simulink model "testSerializedParamsNew"  (R2014a)
settings: Solver=FixedStepDiscrete  StartTime=0.0  StopTime=Inf  FixedStep=0.001  RelTol=1e-3
undefined symbols (not defined in the file or in its folder): SimulinkParameter_TestParam, SimulinkParameter_TestParamPulse, SimulinkParameter_TestParamToggle, SimulinkParameter_TunableTaskControl
libraries: slrtlib x9, dspindex x1
settings Model: SimulationMode=external  BufferReuse=off  Creator=shenoylab  LastModifiedBy=shenoylab
settings SolverCC: EnableConcurrentExecution=on
settings DataIOCC: SignalLoggingSaveFormat=ModelDataLogs
settings OptimizationCC: BlockReduction=off  OptimizeBlockIOStorage=off  BufferReuse=off  GlobalBufferReuse=off  ExpressionFolding=off  LocalBlockOutputs=off
settings DebuggingCC: MultiTaskDSMMsg=warning  MultiTaskCondExecSysMsg=none  StateNameClashWarn=warning
settings HardwareCC: ProdIntDivRoundTo=Zero  ProdEndianess=LittleEndian  ProdHWDeviceType=Generic->32-bit x86 compatible
settings RTWCC: SystemTargetFile=slrt.tlc  TemplateMakefile=slrt_default_tmf  Description=Simulink Real-Time  GenerateReport=on  ProcessScript=slrt_make_rtw_hook  LaunchReport=on  IncludeERTFirstTime=on  RTWCompilerOptimization=On
settings CodeAppCC: MATLABSourceComments=on
settings SimulinkRealTimeCC: GeneratePreprocessorConditionals=Disable all  EnableShiftOperators=on

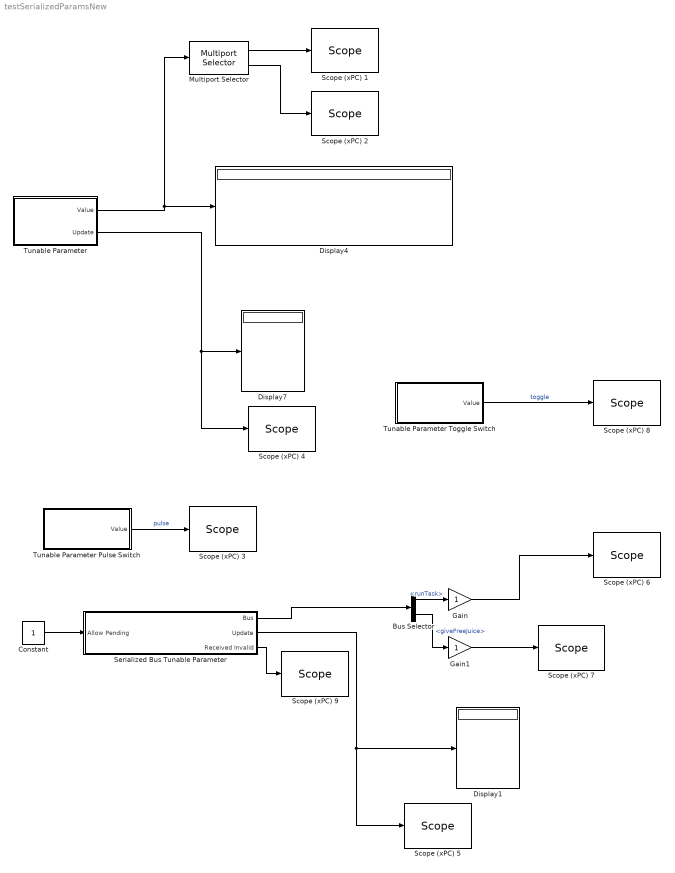
== system testSerializedParamsNew ==
  Bus Selector : BusSelector  OutputSignals=runTask,giveFreeJuice
  Constant : Constant  OutDataTypeStr=uint8
  Display1 : Display
  Display4 : Display
  Display7 : Display
  Gain : Gain  OutDataTypeStr=double
  Gain1 : Gain  OutDataTypeStr=double
  Multiport Selector : dspindex/Multiport Selector  rowsOrCols=Rows  idxCellArray={ 1, 2 }  idxErrMode=Clip Index
  Scope (xPC) 1 : slrtlib/Displays and Logging/Scope   scopeno=1  scopetype=Target  autostart=on  viewmode=Numerical  formatstr='%15.6f'  grid=on  ylimits=[0,0]  nosamples=250  noprepostsamples=0  interleave=1  triggermode=FreeRun  triggersignal=1  trigsignalfromport=off  triggerlevel=0.0  triggerslope=Either  triggerscope=1  triggersample=0  filename=data.dat  mode=Lazy  writesize=512  autorestart=off  dynamicfilemode=off  maxwritefilesize=512*1024^2
  Scope (xPC) 2 : slrtlib/Displays and Logging/Scope   scopeno=2  scopetype=Target  autostart=on  viewmode=Numerical  formatstr='%15.6f'  grid=on  ylimits=[0,0]  nosamples=250  noprepostsamples=0  interleave=1  triggermode=FreeRun  triggersignal=1  trigsignalfromport=off  triggerlevel=0.0  triggerslope=Either  triggerscope=1  triggersample=0  filename=data.dat  mode=Lazy  writesize=512  autorestart=off  dynamicfilemode=off  maxwritefilesize=512*1024^2
  Scope (xPC) 3 : slrtlib/Displays and Logging/Scope   scopeno=3  scopetype=Target  autostart=on  viewmode=Graphical rolling  formatstr='%15.6f'  grid=on  ylimits=[-1,2]  nosamples=500  noprepostsamples=0  interleave=1  triggermode=FreeRun  triggersignal=1  trigsignalfromport=off  triggerlevel=0.0  triggerslope=Either  triggerscope=1  triggersample=0  filename=data.dat  mode=Lazy  writesize=512  autorestart=off  dynamicfilemode=off  maxwritefilesize=512*1024^2
  Scope (xPC) 4 : slrtlib/Displays and Logging/Scope   scopeno=5  scopetype=Target  autostart=on  viewmode=Graphical rolling  formatstr='%15.6f'  grid=on  ylimits=[-1,2]  nosamples=500  noprepostsamples=0  interleave=1  triggermode=FreeRun  triggersignal=1  trigsignalfromport=off  triggerlevel=0.0  triggerslope=Either  triggerscope=1  triggersample=0  filename=data.dat  mode=Lazy  writesize=512  autorestart=off  dynamicfilemode=off  maxwritefilesize=512*1024^2
  Scope (xPC) 5 : slrtlib/Displays and Logging/Scope   scopeno=4  scopetype=Target  autostart=on  viewmode=Graphical rolling  formatstr='%15.6f'  grid=on  ylimits=[-1,2]  nosamples=500  noprepostsamples=0  interleave=1  triggermode=FreeRun  triggersignal=1  trigsignalfromport=off  triggerlevel=0.0  triggerslope=Either  triggerscope=1  triggersample=0  filename=data.dat  mode=Lazy  writesize=512  autorestart=off  dynamicfilemode=off  maxwritefilesize=512*1024^2
  Scope (xPC) 6 : slrtlib/Displays and Logging/Scope   scopeno=6  scopetype=Target  autostart=on  viewmode=Graphical rolling  formatstr='%15.6f'  grid=on  ylimits=[-1,2]  nosamples=250  noprepostsamples=0  interleave=1  triggermode=FreeRun  triggersignal=1  trigsignalfromport=off  triggerlevel=0.0  triggerslope=Either  triggerscope=1  triggersample=0  filename=data.dat  mode=Lazy  writesize=512  autorestart=off  dynamicfilemode=off  maxwritefilesize=512*1024^2
  Scope (xPC) 7 : slrtlib/Displays and Logging/Scope   scopeno=7  scopetype=Target  autostart=on  viewmode=Graphical rolling  formatstr='%15.6f'  grid=on  ylimits=[-1,2]  nosamples=500  noprepostsamples=0  interleave=1  triggermode=FreeRun  triggersignal=1  trigsignalfromport=off  triggerlevel=0.0  triggerslope=Either  triggerscope=1  triggersample=0  filename=data.dat  mode=Lazy  writesize=512  autorestart=off  dynamicfilemode=off  maxwritefilesize=512*1024^2
  Scope (xPC) 8 : slrtlib/Displays and Logging/Scope   scopeno=8  scopetype=Target  autostart=on  viewmode=Graphical rolling  formatstr='%15.6f'  grid=on  ylimits=[-1,2]  nosamples=500  noprepostsamples=0  interleave=1  triggermode=FreeRun  triggersignal=1  trigsignalfromport=off  triggerlevel=0.0  triggerslope=Either  triggerscope=1  triggersample=0  filename=data.dat  mode=Lazy  writesize=512  autorestart=off  dynamicfilemode=off  maxwritefilesize=512*1024^2
  Scope (xPC) 9 : slrtlib/Displays and Logging/Scope   scopeno=9  scopetype=Target  autostart=on  viewmode=Graphical rolling  formatstr='%15.6f'  grid=on  ylimits=[-1,2]  nosamples=500  noprepostsamples=0  interleave=1  triggermode=FreeRun  triggersignal=1  trigsignalfromport=off  triggerlevel=0.0  triggerslope=Either  triggerscope=1  triggersample=0  filename=data.dat  mode=Lazy  writesize=512  autorestart=off  dynamicfilemode=off  maxwritefilesize=512*1024^2
  Serialized Bus Tunable Parameter : Subsystem  AncestorBlock=libBusSerialize/Serialized Bus Tunable Parameter  mask(BusSerialize Tunable Parameter Block){paramName='TunableTaskControl'}
      mask prompts: paramName "Parameter Name"
      mask help: This block provides the value of a tunable Simulink.Parameter into the model. Since tunable parameters with xPC target can only be doubles, the functions BusSerialize.createTunableParameter and BusSerialize.setTunableParameter automatically handle typecasting and update counter insertion, and this block handles update detection, typecasting, and reshaping back to the original form. Currently, variable size parameters are not supported.
      mask init:
      | BusSerialize.maskSerializedBusTunableParameterBlockUpdate(gcb);
      mask Display:
      | port_label('output', 1, paramName);
      | port_label('output', 2, 'Update');
      | port_label('output', 3, 'Received Invalid');
      | port_label('input', 1, 'Allow Pending');
  Tunable Parameter : Subsystem  AncestorBlock=libBusSerialize/Tunable Parameter  mask(BusSerialize Tunable Parameter Block){paramName='TestParam'}
      mask prompts: paramName "Parameter Name"
      mask help: This block provides the value of a tunable Simulink.Parameter into the model. Since tunable parameters with xPC target can only be doubles, the functions BusSerialize.createTunableParameter and BusSerialize.setTunableParameter automatically handle typecasting and update counter insertion, and this block handles update detection, typecasting, and reshaping back to the original form. Currently, variable size parameters are not supported.
      mask init:
      | BusSerialize.maskTunableParameterBlockUpdate(gcb);
      mask Display:
      | port_label('output', 1, paramName)
      | port_label('output', 2, 'Update');
  Tunable Parameter Pulse Switch : Subsystem  AncestorBlock=libBusSerialize/Tunable Parameter Pulse Switch  mask(BusSerialize Tunable Parameter Block){paramName='TestParamPulse'}
      mask prompts: paramName "Parameter Name"
      mask help: This block provides the value of a tunable Simulink.Parameter into the model. Since tunable parameters with xPC target can only be doubles, the functions BusSerialize.createTunableParameter and BusSerialize.setTunableParameter automatically handle typecasting and update counter insertion, and this block handles update detection, typecasting, and reshaping back to the original form. Currently, variable size parameters are not supported.
      mask init:
      | BusSerialize.maskTunableParameterPulseSwitchBlockUpdate(gcb);
      settings: OpenFcn=|
      | paramName = getBlockParamEval(gcb, 'paramName');
      | param = BusSerialize.getTunableParameterReferenceFromName(paramName);
      | param.activatePulseSwitch();
      | 
      | % turn the block green
      | setBlockParam(gcb, 'BackgroundColor', 'green', 'ForegroundColor', 'white');
      | 
      | % wait a bit
      | pause(0.05);
      | 
      | % and set it back to white
      | setBlockParam(gcb, 'BackgroundColor', 'lightBlue', 'ForegroundColor', 'black');
      mask Display: port_label('output', 1, paramName)
  Tunable Parameter Toggle Switch : Subsystem  AncestorBlock=libBusSerialize/Tunable Parameter Toggle Switch  InitFcn=|  mask(BusSerialize Tunable Parameter Block){paramName='TestParamToggle'}
      | if ~isBlockInLibrary(gcb)
      |     paramName = getBlockParamEval(gcb, 'paramName');
      |     param = BusSerialize.getTunableParameterReferenceFromName(paramName);
      |     value = param.value;
      | 
      |     if value
      |         % turn the block green
      |         setBlockParam(gcb, 'BackgroundColor', 'green');  
      |     else
      |         % keep it white
      |         setBlockParam(gcb, 'BackgroundColor', 'lightBlue');
      |     end
      | end
      mask prompts: paramName "Parameter Name"
      mask help:
      | This block provides the value of a tunable Simulink.Parameter into the model. Since tunable parameters with xPC target can only be doubles, the functions BusSerialize.createTunableParameter and BusSerialize.setTunableParameter automatically handle typecasting and update counter insertion, and this block handles update detection, typecasting, and reshaping back to the original form. Currently, variable size parameters are not supported.
      |
      | Use BusSerialize.TunableParameter.create(paramName) to create a parameter with this name.
      mask init:
      | BusSerialize.maskTunableParameterToggleSwitchBlockUpdate(gcb);
      settings: OpenFcn=|
      | if ~isBlockInLibrary(gcb)
      |     paramName = getBlockParamEval(gcb, 'paramName');
      |     param = BusSerialize.getTunableParameterReferenceFromName(paramName);
      |     value = param.toggleSwitch();
      | else
      |     value = uint8(0);
      | end
      | 
      | if value
      |     % turn the block green
      |     setBlockParam(gcb, 'BackgroundColor', 'green');
      | else
      |     % keep it white
      |     setBlockParam(gcb, 'BackgroundColor', 'lightBlue');
      | end
      mask Display: port_label('output', 1, paramName)
  wires:
  Tunable Parameter/2(Update) -> Scope (xPC) 4/1, Display7/1
  Tunable Parameter/1(Value) -> Multiport Selector/1, Display4/1
  Multiport Selector/1 -> Scope (xPC) 1/1
  Multiport Selector/2 -> Scope (xPC) 2/1
  Tunable Parameter Pulse Switch/1(Value) -> Scope (xPC) 3/1  "pulse"
  Constant/1 -> Serialized Bus Tunable Parameter/1(Allow Pending)
  Serialized Bus Tunable Parameter/1(Bus) -> Bus Selector/1
  Serialized Bus Tunable Parameter/2(Update) -> Scope (xPC) 5/1, Display1/1
  Serialized Bus Tunable Parameter/3(Received Invalid) -> Scope (xPC) 9/1
  Bus Selector/1 -> Gain/1  "<runTask>"
  Gain/1 -> Scope (xPC) 6/1
  Bus Selector/2 -> Gain1/1  "<giveFreeJuice>"
  Gain1/1 -> Scope (xPC) 7/1
  Tunable Parameter Toggle Switch/1(Value) -> Scope (xPC) 8/1  "toggle"

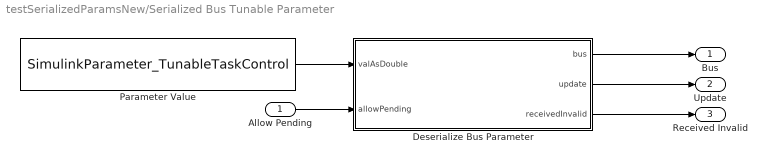
== system testSerializedParamsNew/Serialized Bus Tunable Parameter ==
  Allow Pending : Inport
  Deserialize Bus Parameter : MATLAB Function  TreatAsAtomicUnit=on
  Parameter Value : Constant  Value=SimulinkParameter_TunableTaskControl  OutDataTypeStr=double
  Bus : Outport  PortDimensions=1
  Update : Outport  Port=2  OutDataTypeStr=uint8  PortDimensions=1
  Received Invalid : Outport  Port=3  OutDataTypeStr=uint8  PortDimensions=1
  wires:
  Parameter Value/1 -> Deserialize Bus Parameter/1(valAsDouble)
  Allow Pending/1 -> Deserialize Bus Parameter/2(allowPending)
  Deserialize Bus Parameter/3(receivedInvalid) -> Received Invalid/1
  Deserialize Bus Parameter/1(bus) -> Bus/1
  Deserialize Bus Parameter/2(update) -> Update/1

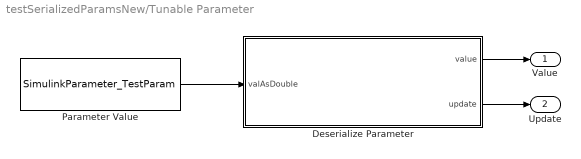
== system testSerializedParamsNew/Tunable Parameter ==
  Deserialize Parameter : MATLAB Function  TreatAsAtomicUnit=on
  Parameter Value : Constant  Value=SimulinkParameter_TestParam  OutDataTypeStr=double
  Value : Outport
  Update : Outport  Port=2
  wires:
  Parameter Value/1 -> Deserialize Parameter/1(valAsDouble)
  Deserialize Parameter/2(update) -> Update/1
  Deserialize Parameter/1(value) -> Value/1

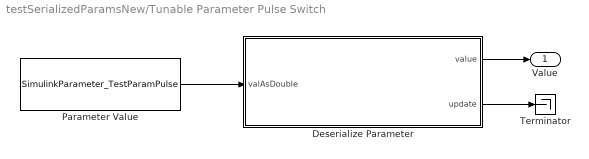
== system testSerializedParamsNew/Tunable Parameter Pulse Switch ==
  Deserialize Parameter : MATLAB Function  TreatAsAtomicUnit=on
  Parameter Value : Constant  Value=SimulinkParameter_TestParamPulse  OutDataTypeStr=double
  Terminator : Terminator
  Value : Outport  OutDataTypeStr=uint8  PortDimensions=1
  wires:
  Parameter Value/1 -> Deserialize Parameter/1(valAsDouble)
  Deserialize Parameter/2(update) -> Terminator/1
  Deserialize Parameter/1(value) -> Value/1

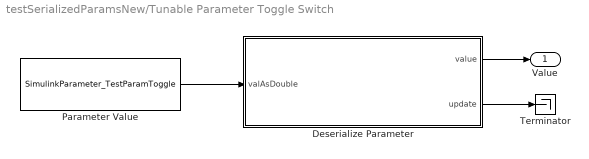
== system testSerializedParamsNew/Tunable Parameter Toggle Switch ==
  Deserialize Parameter : MATLAB Function  TreatAsAtomicUnit=on
  Parameter Value : Constant  Value=SimulinkParameter_TestParamToggle  OutDataTypeStr=double
  Terminator : Terminator
  Value : Outport  OutDataTypeStr=uint8  PortDimensions=1
  wires:
  Parameter Value/1 -> Deserialize Parameter/1(valAsDouble)
  Deserialize Parameter/2(update) -> Terminator/1
  Deserialize Parameter/1(value) -> Value/1

== matlab function testSerializedParamsNew/Tunable Parameter/Deserialize Parameter ==
  data: valAsDouble input double; value output uint16 size=[2 2]; update output uint8 size=1
function [value, update] = deserializeParameter(valAsDouble)
%#codegen

valAsBytes = typecast(valAsDouble, 'uint8');

% check for whether counter has been incremented
thisCounter = valAsBytes(1);
persistent pLastCounter;
if isempty(pLastCounter)
    pLastCounter = thisCounter;
end
if pLastCounter ~= thisCounter
    update = uint8(1);
    pLastCounter = thisCounter;
else
    update = uint8(0);
end

% typecast and reshape the value
value = reshape(typecast(valAsBytes(double(2):double(9)), 'uint16'), [2 2]);

== matlab function testSerializedParamsNew/Tunable Parameter Pulse Switch/Deserialize Parameter ==
  data: valAsDouble input double; value output uint8 size=[1 1]; update output uint8 size=1
function [value, update] = deserializeParameter(valAsDouble)
%#codegen

valAsBytes = typecast(valAsDouble, 'uint8');

% check for whether counter has been incremented
thisCounter = valAsBytes(1);
persistent pLastCounter;
if isempty(pLastCounter)
    pLastCounter = thisCounter;
end
if pLastCounter ~= thisCounter
    update = uint8(1);
    pLastCounter = thisCounter;
else
    update = uint8(0);
end

% typecast and reshape the value
if update ~= uint8(0)
    value = reshape(typecast(valAsBytes(double(2):double(2)), 'uint8'), [1 1]);
else
    value = uint8(0);
end

== matlab function testSerializedParamsNew/Tunable Parameter Toggle Switch/Deserialize Parameter ==
  data: valAsDouble input double; value output uint8 size=[1 1]; update output uint8 size=1
function [value, update] = deserializeParameter(valAsDouble)
%#codegen

valAsBytes = typecast(valAsDouble, 'uint8');

% check for whether counter has been incremented
thisCounter = valAsBytes(1);
persistent pLastCounter;
if isempty(pLastCounter)
    pLastCounter = thisCounter;
end
if pLastCounter ~= thisCounter
    update = uint8(1);
    pLastCounter = thisCounter;
else
    update = uint8(0);
end

% typecast and reshape the value
value = reshape(typecast(valAsBytes(double(2):double(2)), 'uint8'), [1 1]);

== matlab function testSerializedParamsNew/Serialized Bus Tunable Parameter/Deserialize Bus Parameter ==
  data: valAsDouble input double; bus output Bus: TaskControlBus size=1; update output uint8 size=1; allowPending input uint8 size=1; receivedInvalid output uint8 size=1
function [bus, update, receivedInvalid] = deserializeBusParameter(valAsDouble, allowPending)
%#codegen

    % typecast to bytes
    valAsBytes = typecast(valAsDouble, 'uint8');

    % use the first byte as updateCounter, check for whether counter has been incremented
    thisCounter = valAsBytes(1);
    persistent pLastCounter;
    if isempty(pLastCounter)
        pLastCounter = thisCounter;
    end
    if pLastCounter ~= thisCounter
        recvUpdate = uint8(1);
        pLastCounter = thisCounter;
    else
        recvUpdate = uint8(0);
    end
    startOffset = 2;

    % external cached output for when allowPending 
    persistent pBusOut;
    if isempty(pBusOut)
        pBusOut = initializeBus_TaskControlBus();
    end

    % parse incoming bytes if allowing updates
    receivedInvalid = uint8(0);
    if allowPending
        [bus, valid] = deserializeBus_TaskControlBus(valAsBytes, startOffset);
        if valid
            % update internal cache
            pBusOut = bus;
        else
            % don't update internal cache, output internal cache
            bus = pBusOut;
            receivedInvalid = uint8(1);
            recvUpdate = uint8(0);
        end
    else
        bus = pBusOut;
    end

    % track whether we have a pending update
    persistent pPending;
    if isempty(pPending), pPending = uint8(0); end
    if recvUpdate
        if allowPending
            % update goes out immediately
            update = uint8(1);
            pPending = uint8(0);
        else
            % queue pending update
            update = uint8(0);
            pPending = uint8(1);
        end
    else
        if allowPending
            % release pending
            update = pPending;
            pPending = uint8(0);
        else
            % do nothing
            update = uint8(0);
        end
    end

    % reset fields marked with .resetImmediately immediately after update
    if ~update
        bus.giveFreeJuice = uint8(0);
        bus.resetConditionBlock = uint8(0);

    end
end
